simulink subsystem "ITRF_to_GCRF"  (R2022b)
settings: Solver=VariableStepAuto  StartTime=0.0  StopTime=10.0  RelTol=1e-3
settings Model: Creator=laura  LastModifiedBy=laura

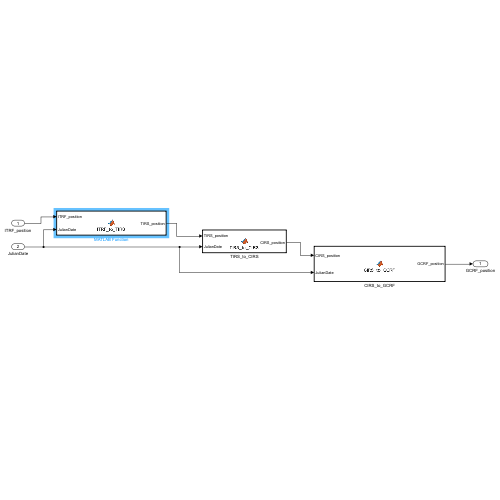
[thumbnail: Simulink's stored preview of the top-level diagram]
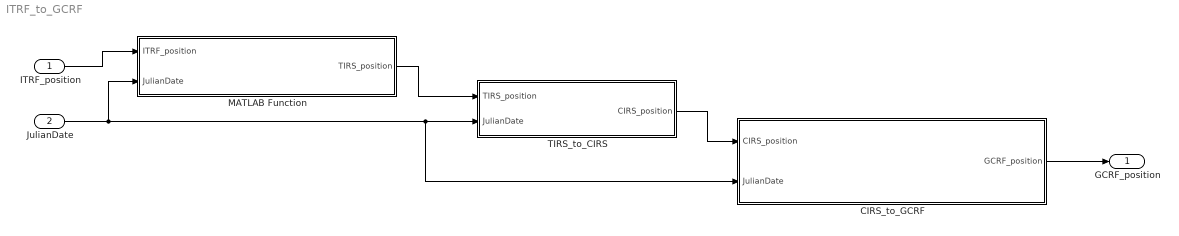
== system ITRF_to_GCRF ==
  ITRF_position : Inport
  JulianDate : Inport  Port=2
  CIRS_to_GCRF : MATLAB Function  TreatAsAtomicUnit=on
  MATLAB Function : MATLAB Function  TreatAsAtomicUnit=on
  TIRS_to_CIRS : MATLAB Function  TreatAsAtomicUnit=on
  GCRF_position : Outport
  wires:
  ITRF_position/1 -> MATLAB Function/1(ITRF_position)
  MATLAB Function/1(TIRS_position) -> TIRS_to_CIRS/1(TIRS_position)
  TIRS_to_CIRS/1(CIRS_position) -> CIRS_to_GCRF/1(CIRS_position)
  JulianDate/1 -> CIRS_to_GCRF/2(JulianDate), TIRS_to_CIRS/2(JulianDate), MATLAB Function/2(JulianDate)
  CIRS_to_GCRF/1(GCRF_position) -> GCRF_position/1

== matlab function ITRF_to_GCRF/MATLAB Function ==
  data: TIRS_position output; ITRF_position input; JulianDate input
function TIRS_position = ITRF_to_TIRS(ITRF_position, JulianDate)

Julian_centuries = (JulianDate - 2451545) / 36525;
s_prime = -0.000047 * 0.00028 * Julian_centuries; % s' is the TIO locator

x_p = -20.7/1000 * 0.00028;     % x_p and y_p are the latest data for the 
y_p = 272.6/1000 * 0.00028;     % International Reference Pole (IRP)

R_x = rotx(y_p);
R_y = roty(x_p); 
R_z = rotz(-s_prime);

TIRS_position = R_z * R_y * R_x * ITRF_position;

== matlab function ITRF_to_GCRF/CIRS_to_GCRF ==
  data: CIRS_position input; GCRF_position output; JulianDate input
function GCRF_position = CIRS_to_GCRF(CIRS_position, JulianDate)

    XValuesTable = readtable("reference_frames\tablea.dat");
    
    % Coordinates of the CIP in the ICRS (figure out calculation later)
    
    rowNumber = 1;

    X = - 0.016617 + 2004.191898*JulianDate - 0.4297829*JulianDate^2 ...
        - 0.19861834 * JulianDate^3 + 0.000007578*JulianDate^4 + 0.0000059285*JulianDate^5;
    
    for i = 1:1306
        a_pi = calculateTrigArgument(XValuesTable{rowNumber, :}, JulianDate);
        X = X + XValuesTable{rowNumber, 4} * sin(a_pi) + XValuesTable{rowNumber, 5} * cos(a_pi);
        rowNumber = rowNumber + 1;
    end    
    
    for i = 1:253
        a_pi = calculateTrigArgument(XValuesTable{rowNumber, :}, JulianDate);
        X = X + (XValuesTable{i, 4} * sin(a_pi) + XValuesTable{i, 5} * cos(a_pi)) * JulianDate;
        rowNumber = rowNumber + 1;
    end

    for i = 1:36
        a_pi = calculateTrigArgument(XValuesTable{rowNumber, :}, JulianDate);
        X = X + (XValuesTable{i, 4} * sin(a_pi) + XValuesTable{i, 5} * cos(a_pi)) * JulianDate^2;
        rowNumber = rowNumber + 1;
    end

    for i = 1:4
        a_pi = calculateTrigArgument(XValuesTable{rowNumber, :}, JulianDate);
        X = X + (XValuesTable{i, 4} * sin(a_pi) + XValuesTable{i, 5} * cos(a_pi)) * JulianDate^3;
        rowNumber = rowNumber + 1;
    end

    a_pi = calculateTrigArgument(XValuesTable{rowNumber, :}, JulianDate);
    X = X + (XValuesTable{i, 4} * sin(a_pi) + XValuesTable{i, 5} * cos(a_pi)) * JulianDate^4;

    % Calculate Y

    YValuesTable = readtable("reference_frames\tableb.dat");
    rowNumber = 1;

    Y = -0.006951 + -0.025896*JulianDate - 22.407274*JulianDate^2 ...
        + 0.00190059* JulianDate^3 + 0.001112526*JulianDate^4 + 0.0000001358*JulianDate^5;
    
    for i = 1:962
        a_pi = calculateTrigArgument(YValuesTable{rowNumber, :}, JulianDate);
        Y = Y + YValuesTable{rowNumber, 4} * sin(a_pi) + YValuesTable{rowNumber, 5} * cos(a_pi);
        rowNumber = rowNumber + 1;
    end    
    
    for i = 1:277
        a_pi = calculateTrigArgument(YValuesTable{rowNumber, :}, JulianDate);
        Y = Y + (YValuesTable{i, 4} * sin(a_pi) + YValuesTable{i, 5} * cos(a_pi)) * JulianDate;
        rowNumber = rowNumber + 1;
    end

    for i = 1:30
        a_pi = calculateTrigArgument(YValuesTable{rowNumber, :}, JulianDate);
       Y = Y + (YValuesTable{i, 4} * sin(a_pi) + YValuesTable{i, 5} * cos(a_pi)) * JulianDate^2;
        rowNumber = rowNumber + 1;
    end

    for i = 1:5
        a_pi = calculateTrigArgument(YValuesTable{rowNumber, :}, JulianDate);
        Y = Y + (YValuesTable{i, 4} * sin(a_pi) + YValuesTable{i, 5} * cos(a_pi)) * JulianDate^3;
        rowNumber = rowNumber + 1;
    end

    a_pi = calculateTrigArgument(YValuesTable{rowNumber, :}, JulianDate);
    Y = Y + (YValuesTable{i, 4} * sin(a_pi) + YValuesTable{i, 5} * cos(a_pi)) * JulianDate^4;
    
    % Calculate s

    sValuesTable = readtable("reference_frames\tablec.dat");
    rowNumber = 1;

    s = -(X*Y)/2;
    s = s + 0.000094 + 0.00380865*JulianDate - 0.00012268*JulianDate^2 ...
        - 0.07257411* JulianDate^3 + 0.00002798*JulianDate^4 + 0.00001562*JulianDate^5;
    
    for i = 1:33
        a_pi = calculateTrigArgument(sValuesTable{rowNumber, :}, JulianDate);
        s = s + sValuesTable{rowNumber, 4} * sin(a_pi) + sValuesTable{rowNumber, 5} * cos(a_pi);
        rowNumber = rowNumber + 1;
    end    
    
    for i = 1:3
        a_pi = calculateTrigArgument(YValuesTable{rowNumber, :}, JulianDate);
        s = s + (sValuesTable{i, 4} * sin(a_pi) + sValuesTable{i, 5} * cos(a_pi)) * JulianDate;
        rowNumber = rowNumber + 1;
    end

    for i = 1:25
        a_pi = calculateTrigArgument(YValuesTable{rowNumber, :}, JulianDate);
        s = s + (sValuesTable{i, 4} * sin(a_pi) + sValuesTable{i, 5} * cos(a_pi)) * JulianDate^2;
        rowNumber = rowNumber + 1;
    end

    for i = 1:4
        a_pi = calculateTrigArgument(YValuesTable{rowNumber, :}, JulianDate);
        s = s + (sValuesTable{i, 4} * sin(a_pi) + sValuesTable{i, 5} * cos(a_pi)) * JulianDate^3;
        rowNumber = rowNumber + 1;
    end

        a_pi = calculateTrigArgument(YValuesTable{rowNumber, :}, JulianDate);
        s = s + (sValuesTable{i, 4} * sin(a_pi) + sValuesTable{i, 5} * cos(a_pi)) * JulianDate^4;


    d = atan(sqrt((X^2 + Y^2) / (1 - X^2 - Y^2)));

    a = 1/(1 + cos(d));
    
    PN = [ (1-a*X^2) (-aXY) (X); (-aXY) (1-aY^2) (Y); (-X) (-Y) (1-a(X^2 +Y^2))];
    R_z = rotz(s);

    GCRF_position = PN*R_z*CIRS_position;

end

function trigArgument = calculateTrigArgument(tableRow, JulianDate)
    trigArgument = 0;
    trigArgument = trigArgument + tableRow{1,6} * (485868.249036 + ...
        1717915923.2178 * JulianDate + 31.8792*JulianDate^2 + 0.051635*JulianDate^3 - ...
        0.00024470 * JulianDate^4);

    trigArgument = trigArgument + tableRow{1,7} * (1287104.79305 + ...
        129596581.048*JulianDate - 0.5532*JulianDate^2 + 0.000136*JulianDate^3 ...
        - 0.00001149*JulianDate^4);
    
    trigArgument = trigArgument + tableRow{1,8} * (335779.526232 + ...
        1739527262.8478*JulianDate - 12.7512*JulianDate^2 - 0.001037*JulianDate^3 + ...
        0.00000417*JulianDate^4);
   
    trigArgument = trigArgument + tableRow{1,9} * (1072260.703 69 + ...
        1602961601.2090*JulianDate - 6.3706*JulianDate^2 + 0.006593*JulianDate^3 - ...
        0.00003169*JulianDate^4);

    trigArgument = trigArgument + tableRow{1,10} * (450160.398036 - ...
        6962890.5431*JulianDate + 7.4722*JulianDate^2 + 0.007702*JulianDate - ...
        0.00005939*JulianDate^4);
    
    trigArgument = trigArgument + tableRow{1,11} * (4.402608842 + 2608.7903141574*JulianDate);
    trigArgument = trigArgument + tableRow{1,12} * (3.176146697 + 1021.3285546211*JulianDate);
    trigArgument = trigArgument + tableRow{1,13} * (1.753470314 + 628.3075849991*JulianDate);
    trigArgument = trigArgument + tableRow{1,14} * (6.203480913 + 334.0612426700*JulianDate);
    trigArgument = trigArgument + tableRow{1,15} * (0.599546497 + 52.9690962641*JulianDate);
    trigArgument = trigArgument + tableRow{1,16} * (0.874016757 + 21.3299104960*JulianDate);
    trigArgument = trigArgument + tableRow{1,17} * (5.481293872 + 7.4781598567*JulianDate);
    trigArgument = trigArgument + tableRow{1,18} * (5.311886287 + 3.8133035638*JulianDate);
    trigArgument = trigArgument + tableRow{1,19} * (0.02438175*JulianDate + 0.00000538691*JulianDate);

end

== matlab function ITRF_to_GCRF/TIRS_to_CIRS ==
  data: TIRS_position input; CIRS_position output; JulianDate input
function CIRS_position = TIRS_to_CIRS(TIRS_position, JulianDate)

Earth_rotation_angle = 2*pi* (0.779057273264 + 1.00273781191135448*(JulianDate - 2451545));

R_z = rotz(-Earth_rotation_angle);

CIRS_position = R_z * TIRS_position;
